simulink model "a2_quad_control_attitude_control"  (R2018b)
settings: Solver=VariableStepAuto  StartTime=0.0  StopTime=50  RelTol=1e-3
undefined symbols (not defined in the file or in its folder): Attitude, AttitudeController, AttitudeTrajectory, drawQuad, P
settings Model: Creator=erics  LastModifiedBy=erics

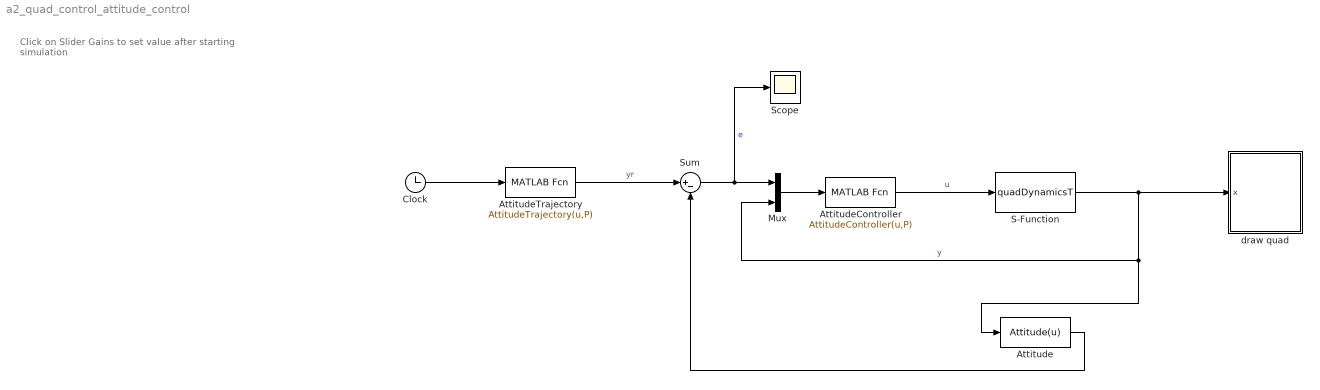
== system a2_quad_control_attitude_control ==
  note: Click on Slider Gains to set value
      | after starting simulation
  Attitude : MATLABFcn  MATLABFcn=Attitude(u)  OutputDimensions=4
  "AttitudeController " : MATLABFcn  MATLABFcn=AttitudeController(u,P)  OutputDimensions=4
  "AttitudeTrajectory " : MATLABFcn  MATLABFcn=AttitudeTrajectory(u,P)  OutputDimensions=4
  Clock : Clock
  Mux : Mux  Inputs=2
  S-Function : S-Function  FunctionName=quadDynamicsT  Parameters=P  SFunctionDeploymentMode=off  EnableBusSupport=off
  Scope : Scope
  Sum : Sum  Inputs=|+-
  draw quad : Subsystem
      mask init:
      | P.courselength = 11;
      | P.coursewidth = 6;
      |     %6ft columns plus four feet of head room
      | P.courseheight = 10;
      | 
      | % quadrotor starting point at 3 ft high and 3 ft in front of the pillars 
      | P.zstart = 0;
      | P.xstart = 0;
      | P.ystart = 0;
      | 
      | % quadrotor dimentions
      |     %2 inches from the center
      | P.boxlength = 1/6;
      | P.boxwidth = P.boxlength;
      |     %4.5 inches from the bottom to the top
      | P.boxheight = 0.375;
      |     %6 inches from box to motor
      | P.armlength = 0.5;
      |     %1/8 inch from center to the side of a rod
      | P.armwidth = 1/96;
      |     %1/4 inch from the top of the box
      | P.armposition = 1/48;
      |     %25*(2)^(1/2)/2 inches from center to perimeter along x and y axis
      | P.perimeter = 1.47;
      |     %perimeter has 3/16 inch width
      | P.periwidth = 1/64;
      | 
      | % pillar dimentions
      |     %6 ft high
      | P.pillarheight = 6;
      |     %5 ft offset;
      | P.pillarposition = 5; 
      |     %5 in radius
      | P.pillarradius = 0.417;
      |     %The adjustment for the none circular pillar
      | P.pillaradd = 0.167;
      |     %The height of each strip on color
      | P.pillarc1 = 0.833; 
      | P.pillarc2 = 0.5;
      mask Display: image(imread('tv.jpg'))
  wires:
  S-Function/1 -> draw quad/1(x), Mux/2, Attitude/1  "y"
  "AttitudeTrajectory "/1 -> Sum/1  "yr"
  "AttitudeController "/1 -> S-Function/1  "u"
  Sum/1 -> Scope/1, Mux/1  "e"
  Clock/1 -> "AttitudeTrajectory "/1
  Attitude/1 -> Sum/2
  Mux/1 -> "AttitudeController "/1

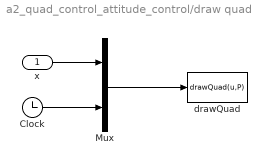
== system a2_quad_control_attitude_control/draw quad ==
  x : Inport
  Clock : Clock
  Mux : Mux  Inputs=2
  drawQuad : MATLABFcn  MATLABFcn=drawQuad(u,P)  OutputDimensions=0  SampleTime=0.1
  wires:
  Mux/1 -> drawQuad/1
  x/1 -> Mux/1
  Clock/1 -> Mux/2
